simulink model "Systeme_Inconnu"  (R2020b)
settings: Solver=VariableStepAuto  StartTime=0.0  StopTime=10  RelTol=1e-3
libraries: pid_lib x1
settings Model: Creator=francesca  LastModifiedBy=Etudiants
settings DataIOCC: ReturnWorkspaceOutputs=off
settings DebuggingCC: ArithmeticOperatorsInVariantConditions=warning
settings SFSimCC: CustomCodeUndefinedFunction=UseInterfaceOnly

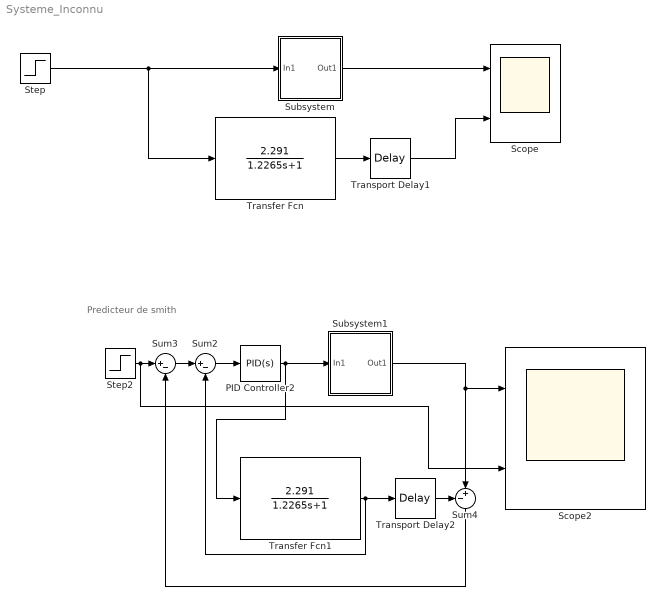
== system Systeme_Inconnu ==
  note: Predicteur de smith
  PID Controller2 : pid_lib/PID Controller  Controller=PID  Form=Ideal  TimeDomain=Continuous-time  UseExternalTs=off  SampleTime=-1  IntegratorMethod=Forward Euler  FilterMethod=Forward Euler  ControllerParametersSource=internal  P=5/2.291  I=1/1.2265  D=0  UseFilter=on  N=100  TunerSelectOption=Transfer Function Based (PID Tuner App)  InitialConditionSource=internal  InitialConditionForIntegrator=0  InitialConditionForFilter=0  DifferentiatorICPrevScaledInput=0  ExternalReset=none  TrackingMode=off  Kt=1  LimitOutput=off  SatLimitsSource=internal  UpperSaturationLimit=inf  LowerSaturationLimit=-inf  LinearizeAsGain=on  AntiWindupMode=none  Kb=1  POutMin=[]  POutMax=[]  IOutMin=[]  IOutMax=[]  DOutMin=[]  DOutMax=[]  NOutMin=[]  NOutMax=[]  SumOutMin=[]  SumOutMax=[]  SaturationOutMin=[]  SaturationOutMax=[]  PParamMin=[]  PParamMax=[]  IParamMin=[]  IParamMax=[]  DParamMin=[]  DParamMax=[]  NParamMin=[]  NParamMax=[]  KbParamMin=[]  KbParamMax=[]  KtParamMin=[]  KtParamMax=[]  KbOutMin=[]  KbOutMax=[]  KtOutMin=[]  KtOutMax=[]  IntegratorOutMin=[]  IntegratorOutMax=[]  FilterOutMin=[]  FilterOutMax=[]  SumI1OutMin=[]  SumI1OutMax=[]  SumI2OutMin=[]  SumI2OutMax=[]  SumI3OutMin=[]  SumI3OutMax=[]  SumI4OutMin=[]  SumI4OutMax=[]  SumDOutMin=[]  SumDOutMax=[]  DifferentiatorOutMin=[]  DifferentiatorOutMax=[]  FilterDiffOutCoefMin=[]  FilterDiffOutCoefMax=[]  ReciprocalOutMin=[]  ReciprocalOutMax=[]  SumDenOutMin=[]  SumDenOutMax=[]  SumNumOutMin=[]  SumNumOutMax=[]  DivideOutMin=[]  DivideOutMax=[]  UdiffTsProdOutMin=[]  UdiffTsProdOutMax=[]  NTsProdOutMin=[]  NTsProdOutMax=[]  UintegralTsProdOutMin=[]  UintegralTsProdOutMax=[]  UngainTsProdOutMin=[]  UngainTsProdOutMax=[]  IntegratorContinuousStateAttributes=''  IntegratorStateMustResolveToSignalObject=off  IntegratorRTWStateStorageClass=Auto  FilterContinuousStateAttributes=''  FilterStateMustResolveToSignalObject=off  FilterRTWStateStorageClass=Auto  ParallelPVariant=Passthrough  IdealPVariant=InternalParameters  IVariant=InternalParameters  DVariant=InternalParameters  IntegratorVariant=Continuous  SatVariant=Disabled  AWVariant=Passthrough  PCopyVariant=Disabled  TRVariant=Disabled  FdbkBlocksVariant=Forward  IdealPFdbkVariant=Disabled  SatFdbkVariant=Disabled  DerivativeFilterVariant=ContFilter  NVariant=InternalParameters  NCopyVariant=Disabled  FilterICVariant=InternalICsFilter  IntegratorICVariant=InternalICs  ExternalResetVariant=Disabled  TRSumVariant=Passthrough  SumFdbkVariant=Disabled  SumVariant=Sum_PID  TsampFilterVariant=InternalTs  TsampNgainVariant=Passthrough  TsampIntegralVariant=Passthrough  ExternalSaturationOutDataTypeStr=Inherit: Same as second input
  Scope : Scope  NumInputPorts=2
  Scope2 : Scope  NumInputPorts=2
  Step : Step  SampleTime=0
  Step2 : Step  SampleTime=0
  Subsystem : Subsystem
  Subsystem1 : Subsystem
  Sum2 : Sum  Inputs=|+-
  Sum3 : Sum  Inputs=|+-
  Sum4 : Sum  Inputs=-+|
  Transfer Fcn : TransferFcn  Numerator=[2.291]  Denominator=[1.2265 1]
  Transfer Fcn1 : TransferFcn  Numerator=[2.291]  Denominator=[1.2265 1]
  Transport Delay1 : TransportDelay  DelayTime=2.1326
  Transport Delay2 : TransportDelay  DelayTime=2.1326
  wires:
  Step/1 -> Transfer Fcn/1, Subsystem/1(In1)
  Subsystem/1(Out1) -> Scope/1
  Sum2/1 -> PID Controller2/1
  Step2/1 -> Scope2/2, Sum3/1
  Sum4/1 -> Sum3/2
  Sum3/1 -> Sum2/1
  Subsystem1/1(Out1) -> Sum4/2, Scope2/1
  PID Controller2/1 -> Transfer Fcn1/1, Subsystem1/1(In1)
  Transfer Fcn/1 -> Transport Delay1/1
  Transport Delay1/1 -> Scope/2
  Transfer Fcn1/1 -> Sum2/2, Transport Delay2/1
  Transport Delay2/1 -> Sum4/1

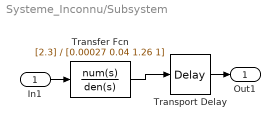
== system Systeme_Inconnu/Subsystem ==
  In1 : Inport
  Transfer Fcn : TransferFcn  Numerator=[2.3]  Denominator=[0.00027 0.04 1.26 1]
  Transport Delay : TransportDelay  DelayTime=2.1  BufferSize=10024
  Out1 : Outport
  wires:
  In1/1 -> Transfer Fcn/1
  Transport Delay/1 -> Out1/1
  Transfer Fcn/1 -> Transport Delay/1

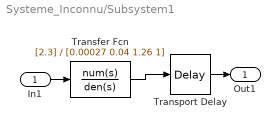
== system Systeme_Inconnu/Subsystem1 ==
  In1 : Inport
  Transfer Fcn : TransferFcn  Numerator=[2.3]  Denominator=[0.00027 0.04 1.26 1]
  Transport Delay : TransportDelay  DelayTime=2.1  BufferSize=10024
  Out1 : Outport
  wires:
  In1/1 -> Transfer Fcn/1
  Transport Delay/1 -> Out1/1
  Transfer Fcn/1 -> Transport Delay/1
